simulink model "test_profile"  (R2020b)
settings: Solver=VariableStepAuto  StartTime=0.0  StopTime=1  MaxStep=1e-3  MinStep=1e-3  RelTol=1e-3
settings Model: Creator=kika  LastModifiedBy=kika

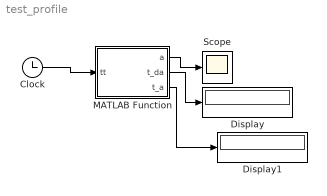
== system test_profile ==
  Clock : Clock
  Display : Display
  Display1 : Display
  MATLAB Function : MATLAB Function  TreatAsAtomicUnit=on
  Scope : Scope
  wires:
  Clock/1 -> MATLAB Function/1(tt)
  MATLAB Function/1(a) -> Scope/1
  MATLAB Function/2(t_da) -> Display/1
  MATLAB Function/3(t_a) -> Display1/1

== matlab function test_profile/MATLAB Function ==
  data: tt input; a output; t_da output; t_a output
function [a, t_da, t_a]= fcn(tt)
     
        v0 = 0.44;
        m_R = 1;
        F_max = 5;
        a_max = F_max / m_R;
        j_max = 100;

        t_a = a_max / j_max;
        t_da = v0 / a_max + t_a;

        a = 0;
        if tt <= t_a
            a = sign(v0) * j_max * tt;
        elseif tt <= (t_da - t_a)
            a = sign(v0) * a_max;
        elseif tt <= t_da
            a = sign(v0) * (j_max * t_da - j_max * tt);
        end
